simulink model "untitled2"  (R2023b)
settings: Solver=ode3  StartTime=0.0  StopTime=inf  RelTol=1e-3
undefined symbols (not defined in the file): a, b1, b2, linear, position, time
libraries: ros2lib x8, fuzblock x1
settings Model: Creator=samee  LastModifiedBy=samee
settings OptimizationCC: EnhancedBackFolding=on  PassReuseOutputArgsAs=Individual arguments  ZeroExternalMemoryAtStartup=off  ZeroInternalMemoryAtStartup=off  MaxStackSize=64  OptimizeBlockOrder=speed  DifferentSizesBufferReuse=on  OptimizationCustomize=off  EfficientTunableParamExpr=on
settings DebuggingCC: ReadBeforeWriteMsg=DisableAll  WriteAfterWriteMsg=DisableAll  WriteAfterReadMsg=DisableAll  MultiTaskDSMMsg=none  ParameterTunabilityLossMsg=error
settings ModelReferenceCC: UpdateModelReferenceTargets=IfOutOfDate
settings SFSimCC: SFSimEcho=off  MATLABDynamicMemAlloc=off  SimTargetLang=C++  GPUAcceleration=on  SimDLTargetLibrary=cudnn
settings RTWCC: Description=Embedded Coder  SystemTargetFile=ert.tlc  HardwareBoard=Robot Operating System 2 (ROS 2)  TLCOptions="-aInlineSetEventsForThisBaseRateFcn=TLC_FALSE -aSuppressMultiTaskScheduler=TLC_FALSE  -aRateBasedStepFcn=0"  GenCodeOnly=on  TemplateMakefile=ert_default_tmf  Toolchain=Colcon Tools  TargetLang=C++
settings CodeAppCC: ForceParamTrailComments=on  IgnoreCustomStorageClasses=off  OperatorAnnotations=on  SimulinkDataObjDesc=on  SFDataObjDesc=on  InsertBlockDesc=on
settings ERTTargetCC: CodeInterfacePackaging=C++ class  SupportContinuousTime=on  RootIOFormat=Structure reference

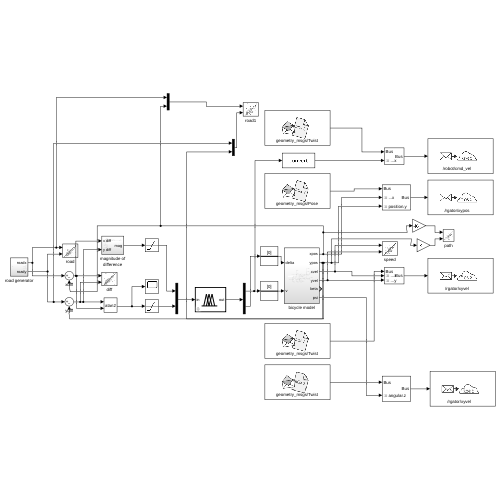
[thumbnail: Simulink's stored preview of the top-level diagram]
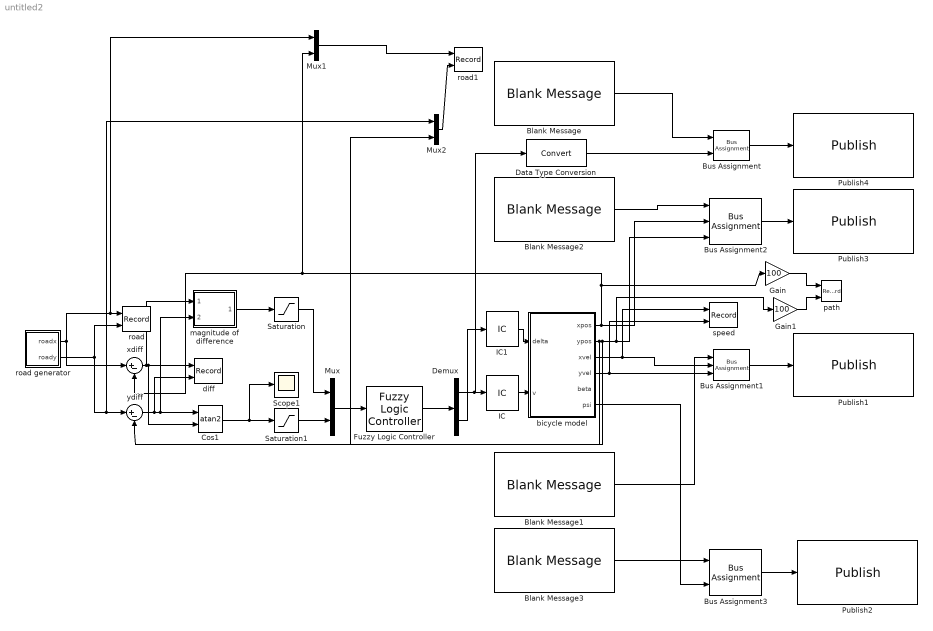
== system untitled2 ==
  Blank Message : ros2lib/Blank Message  messageClass=Message  entityType=geometry_msgs/Twist  messageType=geometry_msgs/Twist  SampleTime=inf
  Blank Message1 : ros2lib/Blank Message  messageClass=Message  entityType=geometry_msgs/Twist  messageType=geometry_msgs/Twist  SampleTime=inf
  Blank Message2 : ros2lib/Blank Message  messageClass=Message  entityType=geometry_msgs/Pose  messageType=geometry_msgs/Pose  SampleTime=inf
  Blank Message3 : ros2lib/Blank Message  messageClass=Message  entityType=geometry_msgs/Twist  messageType=geometry_msgs/Twist  SampleTime=inf
  Bus Assignment : BusAssignment  AssignedSignals=linear.x
  Bus Assignment1 : BusAssignment  AssignedSignals=linear.x,linear.y
  Bus Assignment2 : BusAssignment  AssignedSignals=position.x,position.y
  Bus Assignment3 : BusAssignment  AssignedSignals=angular.z
  Cos1 : Trigonometry  Operator=atan2
  Data Type Conversion : DataTypeConversion  SaturateOnIntegerOverflow=off  RndMeth=Floor
  Demux : Demux  Outputs=2
  Fuzzy Logic Controller : fuzblock/Fuzzy Logic  Controller  FIS=fismatrix  OutputSampleNumber=101  DataType=double  FuzzifiedInputs=off  RuleFiringStrengths=off  RuleOutputs=off  AggregatedOutputs=off  SimulateUsing=Interpreted execution  OutOfRangeInputValueMessage=warning  NoRuleFiredMessage=warning  EmptyOutputFuzzySetMessage=warning
  Gain : Gain  Gain=100
  Gain1 : Gain  Gain=100
  IC : InitialCondition  Value=0
  IC1 : InitialCondition  Value=0
  Mux : Mux  Inputs=2
  Mux1 : Mux  Inputs=2
  Mux2 : Mux  Inputs=2
  Publish1 : ros2lib/Publish  topicSource=Specify your own  topic=/rgator/xyvel  messageType=geometry_msgs/Twist  QOSHistory=Keep last  QOSDepth=1  QOSReliability=Reliable  QOSDurability=Volatile
  Publish2 : ros2lib/Publish  topicSource=Specify your own  topic=/rgator/xyvel  messageType=geometry_msgs/Twist  QOSHistory=Keep last  QOSDepth=1  QOSReliability=Reliable  QOSDurability=Volatile
  Publish3 : ros2lib/Publish  topicSource=Specify your own  topic=/rgator/xypos  messageType=geometry_msgs/Pose  QOSHistory=Keep last  QOSDepth=1  QOSReliability=Reliable  QOSDurability=Volatile
  Publish4 : ros2lib/Publish  topicSource=Specify your own  topic=/robot/cmd_vel  messageType=geometry_msgs/Twist  QOSHistory=Keep last  QOSDepth=1  QOSReliability=Reliable  QOSDurability=Volatile
  Saturation : Saturate  UpperLimit=100  LowerLimit=0  LinearizeAsGain=off
  Saturation1 : Saturate  UpperLimit=1  LowerLimit=-1
  Scope1 : Scope
  bicycle model : Subsystem
  diff : Record  FileSettingsInternal="{\"entries\":[{\"content\":{\"excelSettings\":{\"content\":{},\"type\":\"Streamout.ExcelSettings\"}},\"type\":\"Streamout.FileSettingStorage\",\"uuid\":\"\"}],\"packageUris\":[\"http:\\/\\/schema.mathworks.com\\/mf0\\/streamout_blocks\\/R2020a\"],\"version\":\"1.0\"}"  Layout=[1 1]  SignalsInternal="{\"entries\":[{\"content\":{\"signals\":[{\"content\":{\"blockPath\":[],\"dimensions\":[1],\"domain\":\"\",\"lineColor\":\"#edb120\",\"plots\":[1],\"port\":1,\"sid\":[\"\"],\"signalID\":61,\"signalName\":\"xdiff\"},\"type\":\"RecordBlkView.Signal\",\"uuid\":\"\"},{\"content\":{\"blockPath\":[],\"dimensions\":[1],\"domain\":\"\",\"lineColor\":\"#7e2f8e\",\"plots\":[1],\"port\":2,\"sid\":[\"\"],\"signalID\":65,\"signalName\":\"ydiff\"},\"type\":\"RecordBlkView.Signal\",\"uuid\":\"\"}]},\"type\":\"RecordBlkView.InputSignals\",\"uuid\":\"\"}],\"packageUris\":[\"http:\\/\\/schema.mathworks.com\\/mf0\\/streamout_blocks\\/R2020a\"],\"version\":\"1.0\"}"  VisualizationBindings="{\"xyplotplugin\":{\"info\":[{\"series\":[{\"bindingParametersList\":[{\"parameter\":\"X-Axis\",\"signalID\":61,\"signalName\":\"xdiff\"},{\"parameter\":\"Y-Axis\",\"signalID\":65,\"signalName\":\"ydiff\"}],\"seriesID\":2994}],\"subplotID\":1}]}}"  CompatibilityTag=XY
  magnitude of difference : Subsystem
  path : Record  FileSettingsInternal="{\"entries\":[{\"content\":{\"excelSettings\":{\"content\":{},\"type\":\"Streamout.ExcelSettings\"}},\"type\":\"Streamout.FileSettingStorage\",\"uuid\":\"\"}],\"packageUris\":[\"http:\\/\\/schema.mathworks.com\\/mf0\\/streamout_blocks\\/R2020a\"],\"version\":\"1.0\"}"  Layout=[1 1]  SignalsInternal="{\"entries\":[{\"content\":{\"signals\":[{\"content\":{\"blockPath\":[],\"dimensions\":[1],\"domain\":\"\",\"lineColor\":\"#77ac30\",\"plots\":[1],\"port\":1,\"sid\":[\"\"],\"signalID\":69,\"signalName\":\"Gain\"},\"type\":\"RecordBlkView.Signal\",\"uuid\":\"\"},{\"content\":{\"blockPath\":[],\"dimensions\":[1],\"domain\":\"\",\"lineColor\":\"#4dbeee\",\"plots\":[1],\"port\":2,\"sid\":[\"\"],\"signalID\":73,\"signalName\":\"Gain1\"},\"type\":\"RecordBlkView.Signal\",\"uuid\":\"\"}]},\"type\":\"RecordBlkView.InputSignals\",\"uuid\":\"\"}],\"packageUris\":[\"http:\\/\\/schema.mathworks.com\\/mf0\\/streamout_blocks\\/R2020a\"],\"version\":\"1.0\"}"  VisualizationBindings="{\"xyplotplugin\":{\"info\":[{\"series\":[{\"bindingParametersList\":[{\"parameter\":\"X-Axis\",\"signalID\":69,\"signalName\":\"Gain\"},{\"parameter\":\"Y-Axis\",\"signalID\":73,\"signalName\":\"Gain1\"}],\"seriesID\":32254}],\"subplotID\":1}]}}"  CompatibilityTag=XY
  road : Record  FileSettingsInternal="{\"entries\":[{\"content\":{\"excelSettings\":{\"content\":{},\"type\":\"Streamout.ExcelSettings\"}},\"type\":\"Streamout.FileSettingStorage\",\"uuid\":\"\"}],\"packageUris\":[\"http:\\/\\/schema.mathworks.com\\/mf0\\/streamout_blocks\\/R2020a\"],\"version\":\"1.0\"}"  Layout=[1 1]  SignalsInternal="{\"entries\":[{\"content\":{\"signals\":[{\"content\":{\"blockPath\":[],\"dimensions\":[1],\"domain\":\"\",\"lineColor\":\"#a2142f\",\"plots\":[1],\"port\":1,\"sid\":[\"\"],\"signalID\":77,\"signalName\":\"road generator:1\"},\"type\":\"RecordBlkView.Signal\",\"uuid\":\"\"},{\"content\":{\"blockPath\":[],\"dimensions\":[1],\"domain\":\"\",\"lineColor\":\"#139fff\",\"plots\":[1],\"port\":2,\"sid\":[\"\"],\"signalID\":81,\"signalName\":\"road generator:2\"},\"type\":\"RecordBlkView.Signal\",\"uuid\":\"\"}]},\"type\":\"RecordBlkView.InputSignals\",\"uuid\":\"\"}],\"packageUris\":[\"http:\\/\\/schema.mathworks.com\\/mf0\\/streamout_blocks\\/R2020a\"],\"version\":\"1.0\"}"  VisualizationBindings="{\"xyplotplugin\":{\"info\":[{\"series\":[{\"bindingParametersList\":[{\"parameter\":\"X-Axis\",\"signalID\":77,\"signalName\":\"road generator:1\"},{\"parameter\":\"Y-Axis\",\"signalID\":81,\"signalName\":\"road generator:2\"}],\"seriesID\":59637}],\"subplotID\":1}]}}"  CompatibilityTag=XY
  road generator : Subsystem
  road1 : Record  FileSettingsInternal="{\"entries\":[{\"content\":{\"excelSettings\":{\"content\":{},\"type\":\"Streamout.ExcelSettings\"}},\"type\":\"Streamout.FileSettingStorage\",\"uuid\":\"\"}],\"packageUris\":[\"http:\\/\\/schema.mathworks.com\\/mf0\\/streamout_blocks\\/R2020a\"],\"version\":\"1.0\"}"  Layout=[1 1]  SignalsInternal="{\"entries\":[{\"content\":{\"signals\":[{\"content\":{\"blockPath\":[],\"dimensions\":[2],\"domain\":\"\",\"hasChildren\":true,\"lineColor\":\"#a2142f\",\"port\":1,\"sid\":[\"\"],\"signalID\":85,\"signalName\":\"Mux1\"},\"type\":\"RecordBlkView.Signal\",\"uuid\":\"\"},{\"content\":{\"blockPath\":[],\"channel\":[1],\"dimensions\":[2],\"domain\":\"\",\"lineColor\":\"#139fff\",\"parentID\":85,\"plots\":[1],\"port\":1,\"sid\":[\"\"],\"signalID\":86,\"signalName\":\"Mux1\"},\"type\":\"RecordBlkView.Signal\",\"uuid\":\"\"},{\"content\":{\"blockPath\":[],\"dimensions\":[2],\"domain\":\"\",\"hasChildren\":true,\"lineColor\":\"#ff6929\",\"port\":2,\"sid\":[\"\"],\"signalID\":90,\"signalName\":\"Mux2\"},\"type\":\"RecordBlkView.Signal\",\"uuid\":\"\"},{\"content\":{\"blockPath\":[],\"channel\":[1],\"dimensions\":[2],\"domain\":\"\",\"lineColor\":\"#b746ff\",\"parentID\":90,\"plots\":[1],\"port\":2,\"sid\":[\"\"],\"signalID\":91,\"signalName\":\"Mux2\"},\"type\":\"RecordBlkView.Signal\",\"uuid\":\"\"},{\"content\":{\"blockPath\":[],\"channel\":[2],\"dimensions\":[2],\"domain\":\"\",\"lineColor\":\"#fe330a\",\"parentID\":85,\"plots\":[1],\"port\":1,\"sid\":[\"\"],\"signalID\":103,\"signalName\":\"Mux1\"},\"type\":\"RecordBlkView.Signal\",\"uuid\":\"\"},{\"content\":{\"blockPath\":[],\"channel\":[2],\"dimensions\":[2],\"domain\":\"\",\"lineColor\":\"#22b573\",\"parentID\":90,\"plots\":[1],\"port\":2,\"sid\":[\"\"],\"signalID\":104,\"signalName\":\"Mux2\"},\"type\":\"RecordBlkView.Signal\",\"uuid\":\"\"}]},\"type\":\"RecordBlkView.InputSignals\",\"uuid\":\"\"}],\"packageUris\":[\"http:\\/\\/schema.mathworks.com\\/mf0\\/streamout_blocks\\/R2020a\"],\"version\":\"1.0\"}"  VisualizationBindings="{\"xyplotplugin\":{\"info\":[{\"series\":[{\"bindingParametersList\":[{\"parameter\":\"X-Axis\",\"signalID\":103,\"signalName\":\"Mux1(2)\"},{\"parameter\":\"Y-Axis\",\"signalID\":91,\"signalName\":\"Mux2(1)\"}],\"seriesID\":52058},{\"bindingParametersList\":[{\"parameter\":\"Y-Axis\",\"signalID\":104,\"signalName\":\"Mux2(2)\"},{\"parameter\":\"X-Axis\",\"signalID\":86,\"signalName\":\"Mux1(1)\"}],\"seriesID\":60537}],\"subplotID\":1}]}}"  CompatibilityTag=XY
  speed : Record  FileSettingsInternal="{\"entries\":[{\"content\":{\"excelSettings\":{\"content\":{},\"type\":\"Streamout.ExcelSettings\"}},\"type\":\"Streamout.FileSettingStorage\",\"uuid\":\"\"}],\"packageUris\":[\"http:\\/\\/schema.mathworks.com\\/mf0\\/streamout_blocks\\/R2020a\"],\"version\":\"1.0\"}"  Layout=[1 1]  SignalsInternal="{\"entries\":[{\"content\":{\"signals\":[{\"content\":{\"blockPath\":[],\"dimensions\":[1],\"domain\":\"\",\"lineColor\":\"#ff6929\",\"plots\":[1],\"port\":1,\"sid\":[\"\"],\"signalID\":95,\"signalName\":\"bicycle model:3\"},\"type\":\"RecordBlkView.Signal\",\"uuid\":\"\"},{\"content\":{\"blockPath\":[],\"dimensions\":[1],\"domain\":\"\",\"lineColor\":\"#b746ff\",\"plots\":[1],\"port\":2,\"sid\":[\"\"],\"signalID\":99,\"signalName\":\"bicycle model:4\"},\"type\":\"RecordBlkView.Signal\",\"uuid\":\"\"}]},\"type\":\"RecordBlkView.InputSignals\",\"uuid\":\"\"}],\"packageUris\":[\"http:\\/\\/schema.mathworks.com\\/mf0\\/streamout_blocks\\/R2020a\"],\"version\":\"1.0\"}"  VisualizationBindings="{\"xyplotplugin\":{\"info\":[{\"series\":[{\"bindingParametersList\":[{\"parameter\":\"X-Axis\",\"signalID\":95,\"signalName\":\"bicycle model:3\"},{\"parameter\":\"Y-Axis\",\"signalID\":99,\"signalName\":\"bicycle model:4\"}],\"seriesID\":38694}],\"subplotID\":1}]}}"  CompatibilityTag=XY
  xdiff : Sum  Inputs=|+-
  ydiff : Sum  Inputs=|+-
  wires:
  Bus Assignment1/1 -> Publish1/1
  Bus Assignment2/1 -> Publish3/1
  Blank Message3/1 -> Bus Assignment3/1
  bicycle model/6(psi) -> Bus Assignment3/2
  bicycle model/3(xvel) -> Bus Assignment1/2, speed/1
  bicycle model/2(ypos) -> Mux2/2, Gain1/1, Bus Assignment2/3, ydiff/2
  Blank Message2/1 -> Bus Assignment2/1
  Data Type Conversion/1 -> Bus Assignment/2
  bicycle model/4(yvel) -> speed/2, Bus Assignment1/3
  road generator/2(roady) -> Mux2/1, ydiff/1, road/2
  xdiff/1 -> diff/1, Cos1/2, magnitude of difference/1(x diff)
  bicycle model/1(xpos) -> Mux1/2, xdiff/2, Gain/1, Bus Assignment2/2
  Cos1/1 -> Scope1/1, Saturation1/1
  Blank Message1/1 -> Bus Assignment1/1
  road generator/1(roadx) -> xdiff/1, Mux1/1, road/1
  Saturation/1 -> Mux/1
  Saturation1/1 -> Mux/2
  magnitude of difference/1(mag) -> Saturation/1
  Demux/1 -> Data Type Conversion/1, IC/1
  Bus Assignment/1 -> Publish4/1
  ydiff/1 -> Cos1/1, magnitude of difference/2(y diff), diff/2
  Mux/1 -> Fuzzy Logic Controller/1
  Fuzzy Logic Controller/1 -> Demux/1
  Blank Message/1 -> Bus Assignment/1
  IC/1 -> bicycle model/2(v)
  Demux/2 -> IC1/1
  IC1/1 -> bicycle model/1(delta)
  Gain1/1 -> path/2
  Gain/1 -> path/1
  Bus Assignment3/1 -> Publish2/1
  Mux1/1 -> road1/1
  Mux2/1 -> road1/2

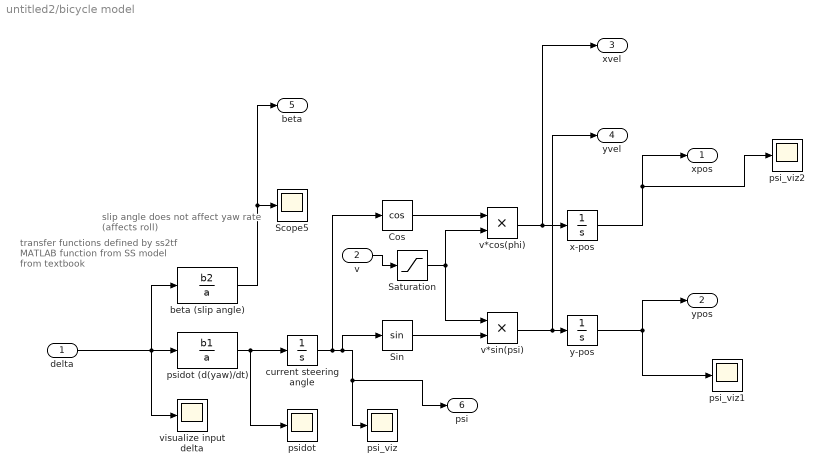
== system untitled2/bicycle model ==
  note: transfer functions defined by ss2tf
      | MATLAB function from SS model
      | from textbook
  note: slip angle does not affect yaw rate
      | (affects roll)
  delta : Inport  OutDataTypeStr=double
  v : Inport  Port=2
  Cos : Trigonometry  Operator=cos
  Saturation : Saturate  UpperLimit=30  LowerLimit=-30
  Scope5 : Scope
  Sin : Trigonometry
  beta (slip angle) : TransferFcn  Numerator=b2  Denominator=a  ContinuousStateAttributes='beta'
  current steering angle : Integrator
  psi_viz : Scope
  psi_viz1 : Scope
  psi_viz2 : Scope
  psidot : Scope
  psidot (d(yaw)/dt) : TransferFcn  Numerator=b1  Denominator=a  ParameterTunability=Optimized  ContinuousStateAttributes='psidot'
  v*cos(phi) : Product
  v*sin(psi) : Product
  visualize input delta : Scope
  x-pos : Integrator
  y-pos : Integrator
  xpos : Outport
  ypos : Outport  Port=2
  xvel : Outport  Port=3
  yvel : Outport  Port=4
  beta : Outport  Port=5
  psi : Outport  Port=6
  wires:
  psidot (d(yaw)/dt)/1 -> current steering angle/1, psidot/1
  v*sin(psi)/1 -> yvel/1, y-pos/1
  current steering angle/1 -> psi/1, psi_viz/1, Sin/1, Cos/1
  delta/1 -> visualize input delta/1, beta (slip angle)/1, psidot (d(yaw)/dt)/1
  Sin/1 -> v*sin(psi)/2
  v*cos(phi)/1 -> xvel/1, x-pos/1
  beta (slip angle)/1 -> beta/1, Scope5/1
  Cos/1 -> v*cos(phi)/1
  y-pos/1 -> psi_viz1/1, ypos/1
  x-pos/1 -> psi_viz2/1, xpos/1
  Saturation/1 -> v*sin(psi)/1, v*cos(phi)/2
  v/1 -> Saturation/1

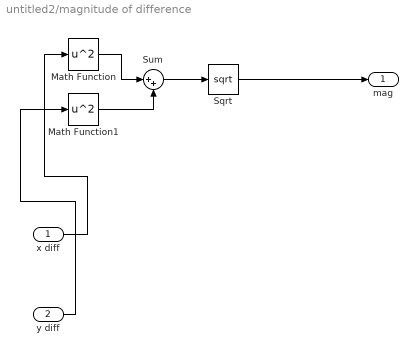
== system untitled2/magnitude of difference ==
  x diff : Inport
  y diff : Inport  Port=2
  Math Function : Math  Operator=square
  Math Function1 : Math  Operator=square
  Sqrt : Sqrt
  Sum : Sum  Inputs=|++
  mag : Outport
  wires:
  Math Function/1 -> Sum/1
  Sum/1 -> Sqrt/1
  Math Function1/1 -> Sum/2
  y diff/1 -> Math Function1/1
  Sqrt/1 -> mag/1
  x diff/1 -> Math Function/1

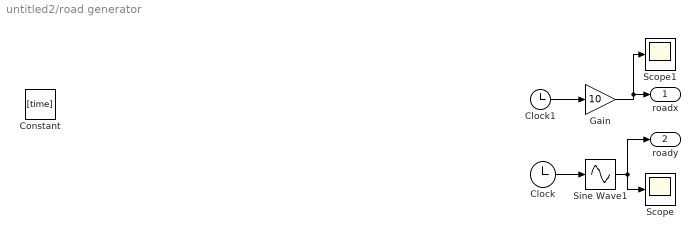
== system untitled2/road generator ==
  Clock : Clock
  Clock1 : Clock
  Constant : Constant  Value=[time]
  Gain : Gain  Gain=10
  Scope : Scope
  Scope1 : Scope
  Sine Wave1 : Sin  TimeSource=Use external signal  Amplitude=10  Frequency=0.05  Phase=1  SampleTime=0
  roadx : Outport
  roady : Outport  Port=2
  wires:
  Clock/1 -> Sine Wave1/1
  Sine Wave1/1 -> Scope/1, roady/1
  Clock1/1 -> Gain/1
  Gain/1 -> Scope1/1, roadx/1
